simulink model "ODE1"  (Simulink 7.8)
settings: Solver=ode45  StartTime=0.0  StopTime=200  RelTol=1e-3
undefined symbols (not defined in the file): a, b, CI1
settings Model: Creator=susana  LastModifiedBy=susana

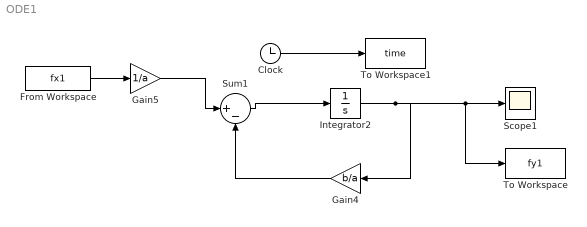
== system ODE1 ==
  Clock : Clock
  From Workspace : FromWorkspace  VariableName=fx1  SampleTime=0
  Gain4 : Gain  Gain=b/a
  Gain5 : Gain  Gain=1/a
  Integrator2 : Integrator  InitialCondition=CI1
  Scope1 : Scope
  Sum1 : Sum  Inputs=|+-
  To Workspace : ToWorkspace  VariableName=fy1  SampleTime=-1  SaveFormat=Array
  To Workspace1 : ToWorkspace  VariableName=time  SampleTime=-1  SaveFormat=Array
  wires:
  Integrator2/1 -> Gain4/1, Scope1/1, To Workspace/1
  Sum1/1 -> Integrator2/1
  Gain5/1 -> Sum1/1
  Gain4/1 -> Sum1/2
  From Workspace/1 -> Gain5/1
  Clock/1 -> To Workspace1/1
